simulink model "FromWorkSpace_interp_extrap_ts"  (R2017b)
settings: Solver=FixedStepDiscrete  StartTime=0.0  StopTime=4  FixedStep=0.100000  RelTol=1e-3
model workspace (MAT data in the model file):
  Var = 0
  matrix_X = timeseries
  matrix_X.Name = 'unnamed'
  matrix_X.DataInfo = tsdata.datametadata
  matrix_X.DataInfo.Interpolation = tsdata.interpolation
  matrix_X.DataInfo.Interpolation.Fhandle : function handle (value not decoded)
  matrix_X.DataInfo.Interpolation.Name = 'linear'
  matrix_X.TimeInfo = tsdata.timemetadata
  matrix_X.TimeInfo.Length = 5
  matrix_X.TimeInfo.DuplicateTimes = 0
  matrix_X.TimeInfo.Time_ = [0; 10; 20; 30; 40]
  matrix_X.TimeInfo.Initialized = 1
  matrix_X.QualityInfo = tsdata.qualmetadata
  matrix_X.Data_ = [1; 2; 3; 4; 5]
settings Model: Creator=hbourbou  LastModifiedBy=hbourbou
settings DataIOCC: SaveFormat=StructureWithTime
settings OptimizationCC: LifeSpan=inf
settings DebuggingCC: SFExecutionAtInitializationDiag=none
settings HardwareCC: ProdBitPerSizeT=32  ProdBitPerPtrDiffT=32  ProdWordSize=32  ProdHWDeviceType=Specified
settings CodeAppCC: StateflowObjectComments=on

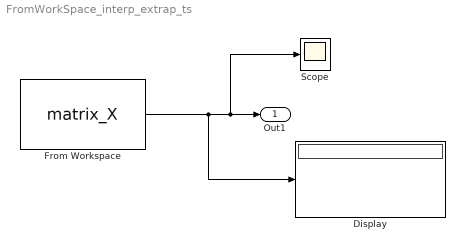
== system FromWorkSpace_interp_extrap_ts ==
  Display : Display
  From Workspace : FromWorkspace  VariableName=matrix_X  SampleTime=.1
  Scope : Scope
  Out1 : Outport
  wires:
  From Workspace/1 -> Display/1, Scope/1, Out1/1
